simulink model "lab04"  (R2023b)
settings: Solver=VariableStepAuto  StartTime=0.0  StopTime=10.0  RelTol=1e-3
undefined symbols (not defined in the file): m
libraries: simulink x2
settings Model: Creator=bissa  LastModifiedBy=bissa

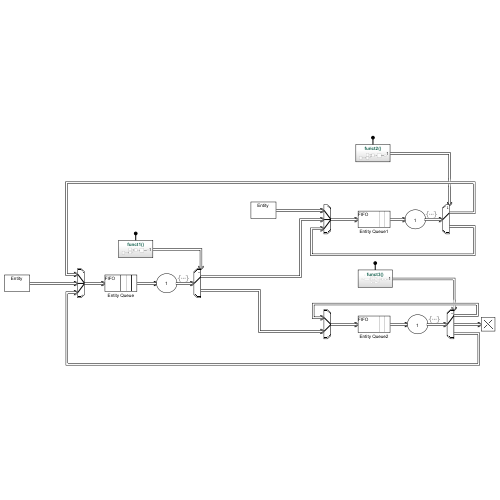
[thumbnail: Simulink's stored preview of the top-level diagram]
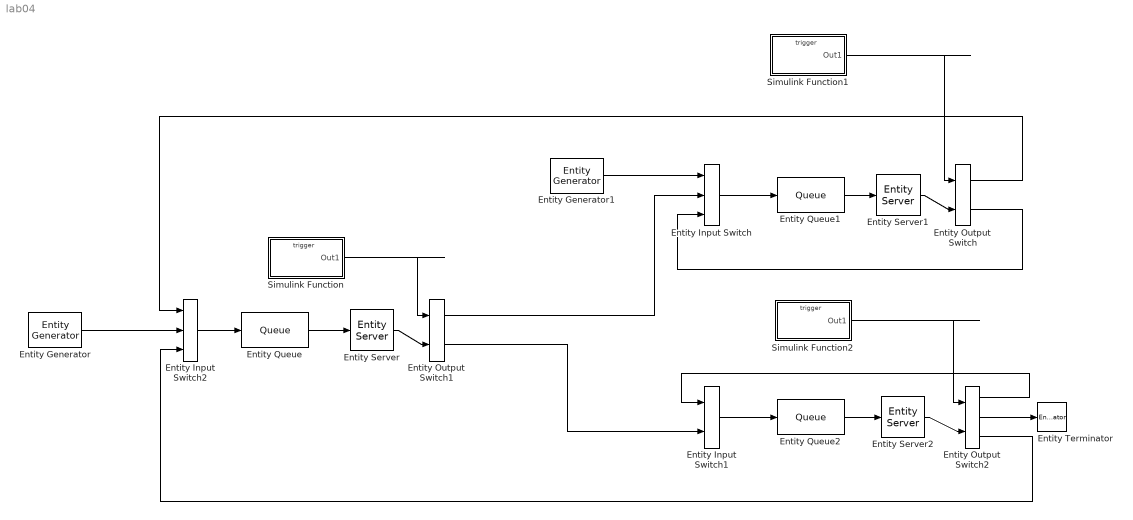
== system lab04 ==
  Entity Input Switch : EntityInputSwitch  InputPortMessageModes=m,m,m  OutputPortMessageModes=m  NumberInputPorts=3
      settings: InputPortMap=u1,u2,u3
  Entity Input Switch1 : EntityInputSwitch  InputPortMessageModes=m,m  OutputPortMessageModes=m
  Entity Input Switch2 : EntityInputSwitch  InputPortMessageModes=m,m,m  OutputPortMessageModes=m  NumberInputPorts=3
      settings: InputPortMap=u1,u2,u3
  Entity Output Switch : EntityOutputSwitch  InputPortMessageModes=m,m  OutputPortMessageModes=m,m  SwitchingCriterion=From control port  SwitchAttributeName=Attribute1
      settings: InputPortMap=u0,u1
  Entity Output Switch1 : EntityOutputSwitch  InputPortMessageModes=m,m  OutputPortMessageModes=m,m  SwitchingCriterion=From control port  SwitchAttributeName=Attribute1
      settings: InputPortMap=u0,u1
  Entity Output Switch2 : EntityOutputSwitch  InputPortMessageModes=m,m  OutputPortMessageModes=m,m,m  NumberOutputPorts=3  SwitchingCriterion=From control port  SwitchAttributeName=Attribute1
      settings: InputPortMap=u0,u1  OutputPortMap=o0,o1,o2
  Entity Generator : EntityGenerator  OutputPortMessageModes=m  TimeSource=MATLAB action  IntergenerationTimeAction=dt = exprnd(1/gamma_1);  EntityType=Structured  EntityTypeName=Entity
  Entity Generator1 : EntityGenerator  OutputPortMessageModes=m  TimeSource=MATLAB action  IntergenerationTimeAction=dt = exprnd(1/gamma_2);  EntityType=Structured  EntityTypeName=Entity
  Entity Queue : Queue  InputPortMessageModes=m  OutputPortMessageModes=m
  Entity Queue1 : Queue  InputPortMessageModes=m  OutputPortMessageModes=m
  Entity Queue2 : Queue  InputPortMessageModes=m  OutputPortMessageModes=m
  Entity Server : EntityServer  InputPortMessageModes=m  OutputPortMessageModes=m  Capacity=1  ServiceTimeSource=MATLAB action  ServiceTimeAction=dt = exprnd(1/mu_1);  ExitAction=funct1
  Entity Server1 : EntityServer  InputPortMessageModes=m  OutputPortMessageModes=m  Capacity=1  ServiceTimeSource=MATLAB action  ServiceTimeAction=dt = exprnd(1/mu_2);  ExitAction=funct2
  Entity Server2 : EntityServer  InputPortMessageModes=m  OutputPortMessageModes=m  Capacity=1  ServiceTimeSource=MATLAB action  ServiceTimeAction=dt = exprnd(1/mu_3);  ExitAction=funct3
  Entity Terminator : EntityTerminator  InputPortMessageModes=m
  Simulink Function : Subsystem  TreatAsAtomicUnit=on
  Simulink Function1 : Subsystem  TreatAsAtomicUnit=on
  Simulink Function2 : Subsystem  TreatAsAtomicUnit=on
  wires:
  Entity Generator1/1 -> Entity Input Switch/1
  Entity Input Switch/1 -> Entity Queue1/1
  Entity Input Switch1/1 -> Entity Queue2/1
  Entity Output Switch1/2 -> Entity Input Switch1/2
  Entity Output Switch1/1 -> Entity Input Switch/2
  Entity Output Switch2/1 -> Entity Input Switch1/1
  Entity Output Switch2/3 -> Entity Input Switch2/3
  Entity Generator/1 -> Entity Input Switch2/2
  Entity Input Switch2/1 -> Entity Queue/1
  Entity Output Switch/1 -> Entity Input Switch2/1
  Entity Output Switch/2 -> Entity Input Switch/3
  Entity Output Switch2/2 -> Entity Terminator/1
  Entity Server/1 -> Entity Output Switch1/2
  Entity Queue/1 -> Entity Server/1
  Entity Queue1/1 -> Entity Server1/1
  Entity Server1/1 -> Entity Output Switch/2
  Entity Queue2/1 -> Entity Server2/1
  Entity Server2/1 -> Entity Output Switch2/2
  Simulink Function/1(Out1) -> Entity Output Switch1/1
  Simulink Function2/1(Out1) -> Entity Output Switch2/1
  Simulink Function1/1(Out1) -> Entity Output Switch/1

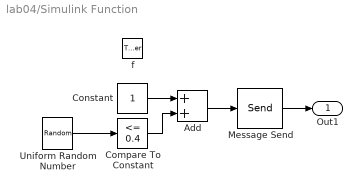
== system lab04/Simulink Function ==
  f : TriggerPort  TriggerType=function-call  IsSimulinkFunction=on  FunctionName=funct1  FunctionVisibility=scoped  VariantControl=(inherit)
  Add : Sum
  Compare To Constant : simulink/Logic and Bit Operations/Compare To Constant  relop=<=  const=0.4  OutDataTypeStr=boolean
  Constant : Constant
  Message Send : Send  OutputPortMessageModes=m
  Uniform Random Number : UniformRandomNumber  Minimum=0  SampleTime=0.1
  Out1 : Outport
  wires:
  Uniform Random Number/1 -> Compare To Constant/1
  Constant/1 -> Add/1
  Compare To Constant/1 -> Add/2
  Add/1 -> Message Send/1
  Message Send/1 -> Out1/1

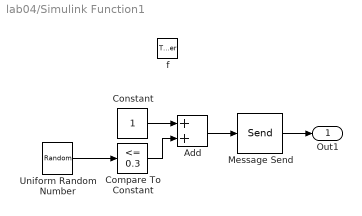
== system lab04/Simulink Function1 ==
  f : TriggerPort  TriggerType=function-call  IsSimulinkFunction=on  FunctionName=funct2  FunctionVisibility=scoped  VariantControl=(inherit)
  Add : Sum
  Compare To Constant : simulink/Logic and Bit Operations/Compare To Constant  relop=<=  const=0.3  OutDataTypeStr=boolean
  Constant : Constant
  Message Send : Send  OutputPortMessageModes=m
  Uniform Random Number : UniformRandomNumber  Minimum=0  SampleTime=0.1
  Out1 : Outport
  wires:
  Message Send/1 -> Out1/1
  Constant/1 -> Add/1
  Add/1 -> Message Send/1
  Uniform Random Number/1 -> Compare To Constant/1
  Compare To Constant/1 -> Add/2

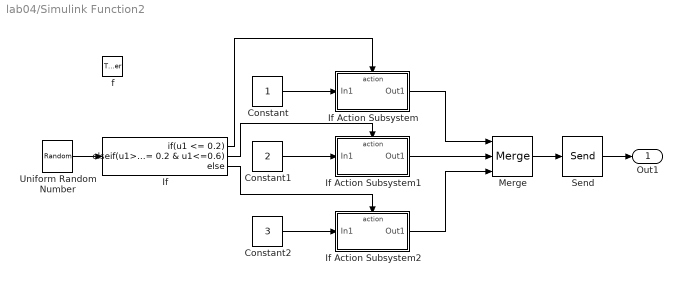
== system lab04/Simulink Function2 ==
  f : TriggerPort  TriggerType=function-call  IsSimulinkFunction=on  FunctionName=funct3  FunctionVisibility=scoped  VariantControl=(inherit)
  Constant : Constant
  Constant1 : Constant  Value=2
  Constant2 : Constant  Value=3
  If : If  IfExpression=u1 <= 0.2  ElseIfExpressions=u1>= 0.2 & u1<=0.6
  If Action Subsystem : Subsystem  TreatAsAtomicUnit=on
  If Action Subsystem1 : Subsystem  TreatAsAtomicUnit=on
  If Action Subsystem2 : Subsystem  TreatAsAtomicUnit=on
  Merge : Merge  Inputs=3
  Send : Send  OutputPortMessageModes=m
  Uniform Random Number : UniformRandomNumber  Minimum=0  SampleTime=0.1
  Out1 : Outport
  wires:
  Uniform Random Number/1 -> If/1
  If Action Subsystem/1(Out1) -> Merge/1
  If/1 -> If Action Subsystem/Action
  If/2 -> If Action Subsystem1/Action
  If/3 -> If Action Subsystem2/Action
  Constant/1 -> If Action Subsystem/1(In1)
  Constant1/1 -> If Action Subsystem1/1(In1)
  Constant2/1 -> If Action Subsystem2/1(In1)
  If Action Subsystem1/1(Out1) -> Merge/2
  If Action Subsystem2/1(Out1) -> Merge/3
  Merge/1 -> Send/1
  Send/1 -> Out1/1

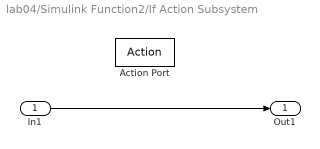
== system lab04/Simulink Function2/If Action Subsystem ==
  In1 : Inport
  Action Port : ActionPort  ActionPortLabel=if(u1 <= 0.2)
  Out1 : Outport
  wires:
  In1/1 -> Out1/1

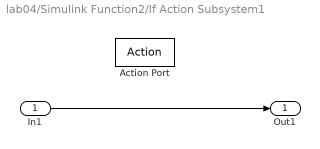
== system lab04/Simulink Function2/If Action Subsystem1 ==
  In1 : Inport
  Action Port : ActionPort  ActionPortLabel=elseif(u2>= 0.2 & u2<=0.6)
  Out1 : Outport
  wires:
  In1/1 -> Out1/1

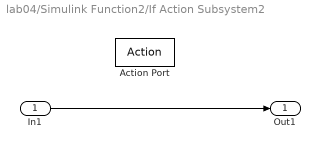
== system lab04/Simulink Function2/If Action Subsystem2 ==
  In1 : Inport
  Action Port : ActionPort  ActionPortLabel=else
  Out1 : Outport
  wires:
  In1/1 -> Out1/1
